simulink model "untitled_restored_from_autosave"  (R2020a)
settings: Solver=VariableStepAuto  StartTime=0.0  StopTime=0.0  RelTol=1e-3
(part 2 of 2)

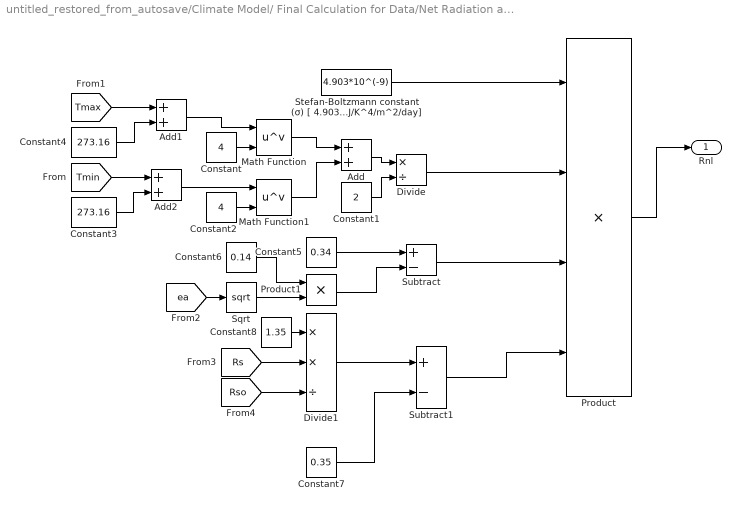
== system untitled_restored_from_autosave/Climate Model/ Final Calculation for Data/Net Radiation at the Crop Surface (Rn) [MJ//m^2//day]/Net Longwave Radiation (Rnl) [MJ//m^2//day] ==
  Add : Sum
  Add1 : Sum
  Add2 : Sum
  Constant : Constant  Value=4
  Constant1 : Constant  Value=2
  Constant2 : Constant  Value=4
  Constant3 : Constant  Value=273.16
  Constant4 : Constant  Value=273.16
  Constant5 : Constant  Value=0.34
  Constant6 : Constant  Value=0.14
  Constant7 : Constant  Value=0.35
  Constant8 : Constant  Value=1.35
  Divide : Product  Inputs=*/
  Divide1 : Product  Inputs=**/
  Math Function : Math  Operator=pow  SaturateOnIntegerOverflow=on
  Math Function1 : Math  Operator=pow  SaturateOnIntegerOverflow=on
  Product : Product  Inputs=4
  Product1 : Product
  Sqrt : Sqrt  SaturateOnIntegerOverflow=on
  Stefan-Boltzmann constant (σ) [ 4.903 10^-9 MJ/K^4/m^2/day] : Constant  Value=4.903*10^(-9)
  Subtract : Sum  Inputs=+-
  Subtract1 : Sum  Inputs=+-
  Rnl : Outport
  wires:
  Product/1 -> Rnl/1
  Stefan-Boltzmann constant (σ) [ 4.903 10^-9 MJ/K^4/m^2/day]/1 -> Product/1
  Constant/1 -> Math Function/2
  Math Function/1 -> Add/1
  Add/1 -> Divide/1
  Divide/1 -> Product/2
  Constant1/1 -> Divide/2
  Math Function1/1 -> Add/2
  Constant2/1 -> Math Function1/2
  Add1/1 -> Math Function/1
  Add2/1 -> Math Function1/1
  Constant3/1 -> Add2/2
  Constant4/1 -> Add1/2
  [Tmin] -> Add2/1
  [Tmax] -> Add1/1
  Subtract/1 -> Product/3
  Constant5/1 -> Subtract/1
  Product1/1 -> Subtract/2
  Constant6/1 -> Product1/1
  Sqrt/1 -> Product1/2
  [ea] -> Sqrt/1
  Subtract1/1 -> Product/4
  Divide1/1 -> Subtract1/1
  Constant7/1 -> Subtract1/2
  Constant8/1 -> Divide1/1
  [Rso] -> Divide1/3
  [Rs] -> Divide1/2

== system untitled_restored_from_autosave/Climate Model/ Final Calculation for Data/Net Radiation at the Crop Surface (Rn) [MJ//m^2//day]/Net Solar//Shortwave Radiation (Rns) [MJ//m^2//day] ==
  Albedo or canopy reflection coefficient for the reference crop (G) : Subsystem
  Constant : Constant
  Product : Product
  Subtract : Sum  Inputs=+-
  Out1 : Outport
  wires:
  Product/1 -> Out1/1
  Constant/1 -> Subtract/1
  Albedo or canopy reflection coefficient for the reference crop (G)/1(Out1) -> Subtract/2
  Subtract/1 -> Product/1
  [Rs] -> Product/2

== system untitled_restored_from_autosave/Climate Model/ Final Calculation for Data/Net Radiation at the Crop Surface (Rn) [MJ//m^2//day]/Solar Radiation (Rs) [MJ//m^2//day] ==
  Actual Duration of Sunlight (n) [hour] : Constant  Value=12
  Angstrom Formula if AI_Rs not avaliable : Subsystem
  Constant : Constant  Value=Ac_Rs
  Constant1 : Constant  Value=5
  Hargreaves Formula if AI_Rs and hour of daylight is not available : Subsystem  mask{kRs=0.16}
      mask prompts: kRs "Adjustment Coefficient"
      mask DialogControl Control2 Prompt: The square root of the temperature difference is closely related to the existing daily solar radiation in a given location. The adjustment coefficient kRs is empirical and differs for 'interior' or 'coastal' regions:
      mask DialogControl Control3 Prompt: · for 'interior' locations, where land mass dominates and air masses are not strongly influenced by a large water body, kRs @ 0.16;
      mask DialogControl Control4 Prompt: · for 'coastal' locations, situated on or adjacent to the coast of a large land mass and where air masses are influenced by a nearby water body, kRs @ 0.19.
  Index Vector : MultiPortSwitch
  Rs : Outport
  wires:
  Constant/1 -> Index Vector/1
  Constant1/1 -> Index Vector/2
  Angstrom Formula if AI_Rs not avaliable/1(Out1) -> Index Vector/3
  Index Vector/1 -> Rs/1
  Hargreaves Formula if AI_Rs and hour of daylight is not available/1(Rs) -> Index Vector/4
  Actual Duration of Sunlight (n) [hour]/1 -> Angstrom Formula if AI_Rs not avaliable/1(In1)

== system untitled_restored_from_autosave/Climate Model/ Final Calculation for Data/Wind Speed/Wind Speed measured at 2m height (u2) [m//s] ==
  uz : Inport
  z : Inport  Port=2
  Constant : Constant  Value=4.87
  Constant1 : Constant  Value=67.8
  Constant2 : Constant  Value=5.42
  Divide : Product  Inputs=**/
  Math Function : Math  Operator=log  SaturateOnIntegerOverflow=on
  Product : Product
  Subtract : Sum  Inputs=+-
  u2 : Outport
  wires:
  uz/1 -> Divide/1
  Constant/1 -> Divide/2
  Math Function/1 -> Divide/3
  z/1 -> Product/2
  Constant1/1 -> Product/1
  Product/1 -> Subtract/1
  Subtract/1 -> Math Function/1
  Constant2/1 -> Subtract/2
  Divide/1 -> u2/1

== system untitled_restored_from_autosave/Estimated Soil Heat Capacity (UC Davis)/Bulk Density (Saxton and Rawls Function) [g//cm^3)/Normal Density (g//cm^3)/Saturated Moisture θS ==
  Constant : Constant  Value=0.097
  Constant1 : Constant  Value=0.043
  Product : Product
  Subtract : Sum  Inputs=++-+
  θ(S-33) : Subsystem
  Out1 : Outport
  wires:
  Subtract/1 -> Out1/1
  [qFC] -> Subtract/1
  Product/1 -> Subtract/3
  Constant/1 -> Product/1
  [PSand] -> Product/2
  Constant1/1 -> Subtract/4
  θ(S-33)/1(Out1) -> Subtract/2

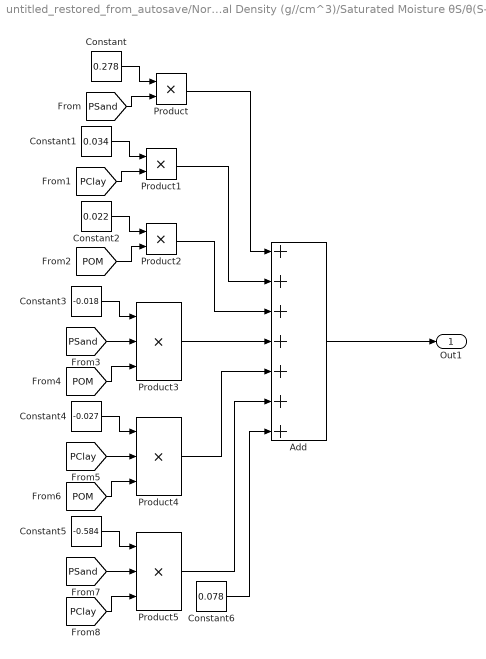
== system untitled_restored_from_autosave/Normal Density (g//cm^3)/Saturated Moisture θS/θ(S-33)/θ(S-33)t ==
  Add : Sum  Inputs=+++++++
  Constant : Constant  Value=0.278
  Constant1 : Constant  Value=0.034
  Constant2 : Constant  Value=0.022
  Constant3 : Constant  Value=-0.018
  Constant4 : Constant  Value=-0.027
  Constant5 : Constant  Value=-0.584
  Constant6 : Constant  Value=0.078
  Product : Product
  Product1 : Product
  Product2 : Product
  Product3 : Product  Inputs=3
  Product4 : Product  Inputs=3
  Product5 : Product  Inputs=3
  Out1 : Outport
  wires:
  Add/1 -> Out1/1
  Constant2/1 -> Product2/1
  [POM] -> Product2/2
  Product1/1 -> Add/2
  Product2/1 -> Add/3
  [PClay] -> Product4/2
  Constant3/1 -> Product3/1
  [POM] -> Product3/3
  [PClay] -> Product1/2
  Constant6/1 -> Add/7
  Product5/1 -> Add/6
  [PClay] -> Product5/3
  Product/1 -> Add/1
  Constant5/1 -> Product5/1
  Constant1/1 -> Product1/1
  Constant/1 -> Product/1
  [POM] -> Product4/3
  Product3/1 -> Add/4
  [PSand] -> Product5/2
  [PSand] -> Product3/2
  Constant4/1 -> Product4/1
  [PSand] -> Product/2
  Product4/1 -> Add/5

== system untitled_restored_from_autosave/Reference Evapotraspiration (ET0) [mm//day]/Actual Vapor Pressure (ea) [kPa]/Derived from Dewpoint Temperature/Saturation Vapor Pressure (eo) ==
  In1 : Inport
  Add : Sum
  Constant : Constant  Value=0.6108
  Constant1 : Constant  Value=17.27
  Constant2 : Constant  Value=237.3
  Divide : Product  Inputs=**/
  Math Function : Math  SaturateOnIntegerOverflow=on
  Product : Product
  Out1 : Outport
  wires:
  Product/1 -> Out1/1
  Constant1/1 -> Divide/1
  In1/1 -> Add/1, Divide/2
  Add/1 -> Divide/3
  Divide/1 -> Math Function/1
  Constant/1 -> Product/1
  Constant2/1 -> Add/2
  Math Function/1 -> Product/2

== system untitled_restored_from_autosave/Reference Evapotraspiration (ET0) [mm//day]/Actual Vapor Pressure (ea) [kPa]/Derived from Psychrometric Data/Saturation Vapor Pressure (eo) ==
  In1 : Inport
  Add : Sum
  Constant : Constant  Value=0.6108
  Constant1 : Constant  Value=17.27
  Constant2 : Constant  Value=237.3
  Divide : Product  Inputs=**/
  Math Function : Math  SaturateOnIntegerOverflow=on
  Product : Product
  Out1 : Outport
  wires:
  Product/1 -> Out1/1
  Constant1/1 -> Divide/1
  In1/1 -> Add/1, Divide/2
  Add/1 -> Divide/3
  Divide/1 -> Math Function/1
  Constant/1 -> Product/1
  Constant2/1 -> Add/2
  Math Function/1 -> Product/2

== system untitled_restored_from_autosave/Reference Evapotraspiration (ET0) [mm//day]/Actual Vapor Pressure (ea) [kPa]/Derived from RHmax & RHmin/Saturation Vapor Pressure (eo) ==
  In1 : Inport
  Add : Sum
  Constant : Constant  Value=0.6108
  Constant1 : Constant  Value=17.27
  Constant2 : Constant  Value=237.3
  Divide : Product  Inputs=**/
  Math Function : Math  SaturateOnIntegerOverflow=on
  Product : Product
  Out1 : Outport
  wires:
  Product/1 -> Out1/1
  Constant1/1 -> Divide/1
  In1/1 -> Add/1, Divide/2
  Add/1 -> Divide/3
  Divide/1 -> Math Function/1
  Constant/1 -> Product/1
  Constant2/1 -> Add/2
  Math Function/1 -> Product/2

== system untitled_restored_from_autosave/Reference Evapotraspiration (ET0) [mm//day]/Actual Vapor Pressure (ea) [kPa]/Derived from RHmax & RHmin/Saturation Vapor Pressure (eo)1 ==
  In1 : Inport
  Add : Sum
  Constant : Constant  Value=0.6108
  Constant1 : Constant  Value=17.27
  Constant2 : Constant  Value=237.3
  Divide : Product  Inputs=**/
  Math Function : Math  SaturateOnIntegerOverflow=on
  Product : Product
  Out1 : Outport
  wires:
  Math Function/1 -> Product/2
  Constant2/1 -> Add/2
  Constant/1 -> Product/1
  Divide/1 -> Math Function/1
  Add/1 -> Divide/3
  In1/1 -> Divide/2, Add/1
  Constant1/1 -> Divide/1
  Product/1 -> Out1/1

== system untitled_restored_from_autosave/Reference Evapotraspiration (ET0) [mm//day]/Actual Vapor Pressure (ea) [kPa]/Derived from RHmax only/Saturation Vapor Pressure (eo) ==
  In1 : Inport
  Add : Sum
  Constant : Constant  Value=0.6108
  Constant1 : Constant  Value=17.27
  Constant2 : Constant  Value=237.3
  Divide : Product  Inputs=**/
  Math Function : Math  SaturateOnIntegerOverflow=on
  Product : Product
  Out1 : Outport
  wires:
  Product/1 -> Out1/1
  Constant1/1 -> Divide/1
  In1/1 -> Add/1, Divide/2
  Add/1 -> Divide/3
  Divide/1 -> Math Function/1
  Constant/1 -> Product/1
  Constant2/1 -> Add/2
  Math Function/1 -> Product/2

== system untitled_restored_from_autosave/Reference Evapotraspiration (ET0) [mm//day]/Actual Vapor Pressure (ea) [kPa]/Derived from RHmean only/Saturation Vapor Pressure (eo) ==
  In1 : Inport
  Add : Sum
  Constant : Constant  Value=0.6108
  Constant1 : Constant  Value=17.27
  Constant2 : Constant  Value=237.3
  Divide : Product  Inputs=**/
  Math Function : Math  SaturateOnIntegerOverflow=on
  Product : Product
  Out1 : Outport
  wires:
  Product/1 -> Out1/1
  Constant1/1 -> Divide/1
  In1/1 -> Add/1, Divide/2
  Add/1 -> Divide/3
  Divide/1 -> Math Function/1
  Constant/1 -> Product/1
  Constant2/1 -> Add/2
  Math Function/1 -> Product/2

== system untitled_restored_from_autosave/Reference Evapotraspiration (ET0) [mm//day]/Actual Vapor Pressure (ea) [kPa]/Derived from RHmean only/Saturation Vapor Pressure (eo)1 ==
  In1 : Inport
  Add : Sum
  Constant : Constant  Value=0.6108
  Constant1 : Constant  Value=17.27
  Constant2 : Constant  Value=237.3
  Divide : Product  Inputs=**/
  Math Function : Math  SaturateOnIntegerOverflow=on
  Product : Product
  Out1 : Outport
  wires:
  Math Function/1 -> Product/2
  Constant2/1 -> Add/2
  Constant/1 -> Product/1
  Divide/1 -> Math Function/1
  Add/1 -> Divide/3
  In1/1 -> Divide/2, Add/1
  Constant1/1 -> Divide/1
  Product/1 -> Out1/1

== system untitled_restored_from_autosave/Soil Data Calculation/Estimated Soil Heat Capacity (UC Davis)/Bulk Density (Saxton and Rawls Function) [g//cm^3)/Normal Density (g//cm^3) ==
  Constant : Constant  Value=2.65
  Constant1 : Constant
  Product : Product
  Saturated Moisture θS : Subsystem
  Subtract : Sum  Inputs=+-
  Out1 : Outport
  wires:
  Product/1 -> Out1/1
  Constant/1 -> Product/2
  Subtract/1 -> Product/1
  Constant1/1 -> Subtract/1
  Saturated Moisture θS/1(Out1) -> Subtract/2

== system untitled_restored_from_autosave/Soil Data Calculation/Estimated Soil Heat Capacity (UC Davis)/Bulk Density (Saxton and Rawls Function) [g//cm^3)/Volum Fraction of Gravel (g//cm^3) ==
  In1 : Inport
  Constant : Constant  Value=2.65
  Constant1 : Constant
  Constant2 : Constant
  Divide : Product  Inputs=*/
  Divide1 : Product  Inputs=*/
  Product : Product
  Product1 : Product
  Subtract : Sum  Inputs=+-
  Subtract1 : Sum  Inputs=+-
  Out1 : Outport
  wires:
  In1/1 -> Divide/1
  [PGravel] -> Product1/1, Product/2
  Constant/1 -> Divide/2
  Divide/1 -> Subtract1/2, Product/1
  Product/1 -> Divide1/1
  Subtract/1 -> Divide1/2
  Constant1/1 -> Subtract/1
  Product1/1 -> Subtract/2
  Subtract1/1 -> Product1/2
  Constant2/1 -> Subtract1/1
  Divide1/1 -> Out1/1

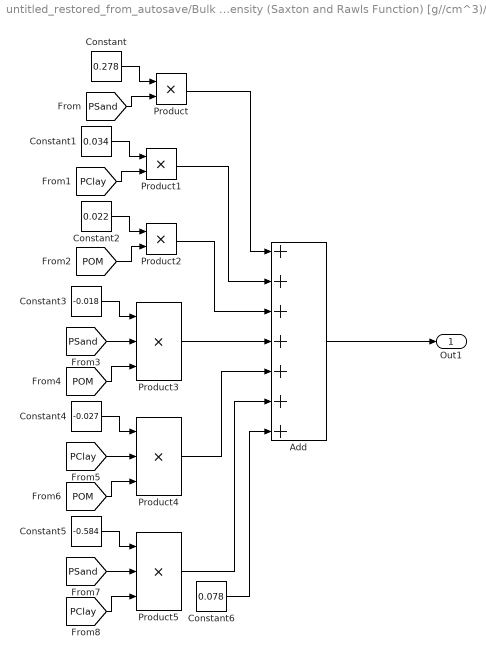
== system untitled_restored_from_autosave/Bulk Density (Saxton and Rawls Function) [g//cm^3)/Normal Density (g//cm^3)/Saturated Moisture θS/θ(S-33)/θ(S-33)t ==
  Add : Sum  Inputs=+++++++
  Constant : Constant  Value=0.278
  Constant1 : Constant  Value=0.034
  Constant2 : Constant  Value=0.022
  Constant3 : Constant  Value=-0.018
  Constant4 : Constant  Value=-0.027
  Constant5 : Constant  Value=-0.584
  Constant6 : Constant  Value=0.078
  Product : Product
  Product1 : Product
  Product2 : Product
  Product3 : Product  Inputs=3
  Product4 : Product  Inputs=3
  Product5 : Product  Inputs=3
  Out1 : Outport
  wires:
  Add/1 -> Out1/1
  Constant2/1 -> Product2/1
  [POM] -> Product2/2
  Product1/1 -> Add/2
  Product2/1 -> Add/3
  [PClay] -> Product4/2
  Constant3/1 -> Product3/1
  [POM] -> Product3/3
  [PClay] -> Product1/2
  Constant6/1 -> Add/7
  Product5/1 -> Add/6
  [PClay] -> Product5/3
  Product/1 -> Add/1
  Constant5/1 -> Product5/1
  Constant1/1 -> Product1/1
  Constant/1 -> Product/1
  [POM] -> Product4/3
  Product3/1 -> Add/4
  [PSand] -> Product5/2
  [PSand] -> Product3/2
  Constant4/1 -> Product4/1
  [PSand] -> Product/2
  Product4/1 -> Add/5

== system untitled_restored_from_autosave/Climate Model/ Final Calculation for Data/Net Radiation at the Crop Surface (Rn) [MJ//m^2//day]/Extraterrestrial Radiation (Ra) [MJ//m^2//day]/Inverse Relative Distance Earth-Sun (dr) ==
  J : Inport
  Add : Sum
  Constant : Constant
  Constant1 : Constant  Value=0.033
  Constant2 : Constant  Value=2*pi
  Divide : Product  Inputs=**/
  Product : Product
  Trigonometric Function : Trigonometry  Operator=cos
  dr : Outport
  wires:
  Add/1 -> dr/1
  Constant/1 -> Add/1
  Product/1 -> Add/2
  Constant1/1 -> Product/1
  Trigonometric Function/1 -> Product/2
  Divide/1 -> Trigonometric Function/1
  Constant2/1 -> Divide/1
  [DinYear] -> Divide/3
  J/1 -> Divide/2

== system untitled_restored_from_autosave/Climate Model/ Final Calculation for Data/Net Radiation at the Crop Surface (Rn) [MJ//m^2//day]/Extraterrestrial Radiation (Ra) [MJ//m^2//day]/Latitude in Radian (φ) [rad] ==
  Add : Sum
  Constant : Constant  Value=pi/180
  Constant1 : Constant  Value=60
  Divide : Product  Inputs=*/
  Product : Product
  φ : Outport
  wires:
  Constant/1 -> Product/1
  Add/1 -> Product/2
  [LatDeg] -> Add/1
  [LatMin] -> Divide/1
  Constant1/1 -> Divide/2
  Divide/1 -> Add/2
  Product/1 -> φ/1

== system untitled_restored_from_autosave/Climate Model/ Final Calculation for Data/Net Radiation at the Crop Surface (Rn) [MJ//m^2//day]/Extraterrestrial Radiation (Ra) [MJ//m^2//day]/Solar Declination in Radian (δ) [rad] ==
  J : Inport
  Constant1 : Constant  Value=0.409
  Constant2 : Constant  Value=2*pi
  Constant4 : Constant  Value=1.39
  Divide : Product  Inputs=**/
  Product : Product
  Subtract : Sum  Inputs=+-
  Trigonometric Function : Trigonometry
  δ : Outport
  wires:
  [DinYear] -> Divide/3
  Product/1 -> δ/1
  Trigonometric Function/1 -> Product/2
  J/1 -> Divide/2
  Constant2/1 -> Divide/1
  Constant1/1 -> Product/1
  Divide/1 -> Subtract/1
  Subtract/1 -> Trigonometric Function/1
  Constant4/1 -> Subtract/2

== system untitled_restored_from_autosave/Climate Model/ Final Calculation for Data/Net Radiation at the Crop Surface (Rn) [MJ//m^2//day]/Extraterrestrial Radiation (Ra) [MJ//m^2//day]/Sunset Hour Angle (Ws) [rad] ==
  Constant : Constant  Value=-1
  Product : Product  Inputs=3
  Trigonometric Function : Trigonometry  Operator=acos
  Trigonometric Function1 : Trigonometry  Operator=tan
  Trigonometric Function2 : Trigonometry  Operator=tan
  Ws : Outport
  wires:
  Trigonometric Function/1 -> Ws/1
  Product/1 -> Trigonometric Function/1
  Constant/1 -> Product/1
  Trigonometric Function1/1 -> Product/2
  Trigonometric Function2/1 -> Product/3
  [LatRad] -> Trigonometric Function1/1
  [SolDec] -> Trigonometric Function2/1

== system untitled_restored_from_autosave/Climate Model/ Final Calculation for Data/Net Radiation at the Crop Surface (Rn) [MJ//m^2//day]/Net Solar//Shortwave Radiation (Rns) [MJ//m^2//day]/Albedo or canopy reflection coefficient for the reference crop (G) ==
  Constant : Constant  Value=0.23
  Out1 : Outport
  wires:
  Constant/1 -> Out1/1

== system untitled_restored_from_autosave/Climate Model/ Final Calculation for Data/Net Radiation at the Crop Surface (Rn) [MJ//m^2//day]/Solar Radiation (Rs) [MJ//m^2//day]/Angstrom Formula if AI_Rs not avaliable ==
  In1 : Inport
  Add : Sum
  Default as : Constant  Value=0.25
  Default bs : Constant  Value=0.50
  Divide : Product  Inputs=**/
  Maximum Daylight Hour (N) [hour] : Subsystem
  Product : Product
  Out1 : Outport
  wires:
  Default as/1 -> Add/1
  Default bs/1 -> Divide/1
  Divide/1 -> Add/2
  In1/1 -> Divide/2
  Add/1 -> Product/1
  Product/1 -> Out1/1
  [Ra] -> Product/2
  Maximum Daylight Hour (N) [hour]/1(N) -> Divide/3

== system untitled_restored_from_autosave/Climate Model/ Final Calculation for Data/Net Radiation at the Crop Surface (Rn) [MJ//m^2//day]/Solar Radiation (Rs) [MJ//m^2//day]/Hargreaves Formula if AI_Rs and hour of daylight is not available ==
  Constant : Constant  Value=kRs
  Product : Product  Inputs=3
  Sqrt : Sqrt  SaturateOnIntegerOverflow=on
  Subtract : Sum  Inputs=+-
  Rs : Outport
  wires:
  Product/1 -> Rs/1
  Constant/1 -> Product/1
  [Ra] -> Product/3
  Sqrt/1 -> Product/2
  Subtract/1 -> Sqrt/1
  [Tmin] -> Subtract/2
  [Tmax] -> Subtract/1

== system untitled_restored_from_autosave/Estimated Soil Heat Capacity (UC Davis)/Bulk Density (Saxton and Rawls Function) [g//cm^3)/Normal Density (g//cm^3)/Saturated Moisture θS/θ(S-33) ==
  Constant : Constant  Value=0.636
  Constant1 : Constant  Value=0.107
  Product : Product
  Subtract : Sum  Inputs=++-
  θ(S-33)t : Subsystem
  Out1 : Outport
  wires:
  θ(S-33)t/1(Out1) -> Product/1, Subtract/1
  Product/1 -> Subtract/2
  Constant/1 -> Product/2
  Constant1/1 -> Subtract/3
  Subtract/1 -> Out1/1

== system untitled_restored_from_autosave/Soil Data Calculation/Estimated Soil Heat Capacity (UC Davis)/Bulk Density (Saxton and Rawls Function) [g//cm^3)/Normal Density (g//cm^3)/Saturated Moisture θS ==
  Constant : Constant  Value=0.097
  Constant1 : Constant  Value=0.043
  Product : Product
  Subtract : Sum  Inputs=++-+
  θ(S-33) : Subsystem
  Out1 : Outport
  wires:
  Subtract/1 -> Out1/1
  [qFC] -> Subtract/1
  Product/1 -> Subtract/3
  Constant/1 -> Product/1
  [PSand] -> Product/2
  Constant1/1 -> Subtract/4
  θ(S-33)/1(Out1) -> Subtract/2

== system untitled_restored_from_autosave/Climate Model/ Final Calculation for Data/Net Radiation at the Crop Surface (Rn) [MJ//m^2//day]/Solar Radiation (Rs) [MJ//m^2//day]/Angstrom Formula if AI_Rs not avaliable/Maximum Daylight Hour (N) [hour] ==
  Constant : Constant  Value=24
  Constant1 : Constant  Value=pi
  Divide : Product  Inputs=**/
  N : Outport
  wires:
  Divide/1 -> N/1
  [Ws] -> Divide/2
  Constant/1 -> Divide/1
  Constant1/1 -> Divide/3

== system untitled_restored_from_autosave/Estimated Soil Heat Capacity (UC Davis)/Bulk Density (Saxton and Rawls Function) [g//cm^3)/Normal Density (g//cm^3)/Saturated Moisture θS/θ(S-33)/θ(S-33)t ==
  Add : Sum  Inputs=+++++++
  Constant : Constant  Value=0.278
  Constant1 : Constant  Value=0.034
  Constant2 : Constant  Value=0.022
  Constant3 : Constant  Value=-0.018
  Constant4 : Constant  Value=-0.027
  Constant5 : Constant  Value=-0.584
  Constant6 : Constant  Value=0.078
  Product : Product
  Product1 : Product
  Product2 : Product
  Product3 : Product  Inputs=3
  Product4 : Product  Inputs=3
  Product5 : Product  Inputs=3
  Out1 : Outport
  wires:
  Add/1 -> Out1/1
  Constant2/1 -> Product2/1
  [POM] -> Product2/2
  Product1/1 -> Add/2
  Product2/1 -> Add/3
  [PClay] -> Product4/2
  Constant3/1 -> Product3/1
  [POM] -> Product3/3
  [PClay] -> Product1/2
  Constant6/1 -> Add/7
  Product5/1 -> Add/6
  [PClay] -> Product5/3
  Product/1 -> Add/1
  Constant5/1 -> Product5/1
  Constant1/1 -> Product1/1
  Constant/1 -> Product/1
  [POM] -> Product4/3
  Product3/1 -> Add/4
  [PSand] -> Product5/2
  [PSand] -> Product3/2
  Constant4/1 -> Product4/1
  [PSand] -> Product/2
  Product4/1 -> Add/5

== system untitled_restored_from_autosave/Soil Data Calculation/Estimated Soil Heat Capacity (UC Davis)/Bulk Density (Saxton and Rawls Function) [g//cm^3)/Normal Density (g//cm^3)/Saturated Moisture θS/θ(S-33) ==
  Constant : Constant  Value=0.636
  Constant1 : Constant  Value=0.107
  Product : Product
  Subtract : Sum  Inputs=++-
  θ(S-33)t : Subsystem
  Out1 : Outport
  wires:
  θ(S-33)t/1(Out1) -> Product/1, Subtract/1
  Product/1 -> Subtract/2
  Constant/1 -> Product/2
  Constant1/1 -> Subtract/3
  Subtract/1 -> Out1/1

== system untitled_restored_from_autosave/Soil Data Calculation/Estimated Soil Heat Capacity (UC Davis)/Bulk Density (Saxton and Rawls Function) [g//cm^3)/Normal Density (g//cm^3)/Saturated Moisture θS/θ(S-33)/θ(S-33)t ==
  Add : Sum  Inputs=+++++++
  Constant : Constant  Value=0.278
  Constant1 : Constant  Value=0.034
  Constant2 : Constant  Value=0.022
  Constant3 : Constant  Value=-0.018
  Constant4 : Constant  Value=-0.027
  Constant5 : Constant  Value=-0.584
  Constant6 : Constant  Value=0.078
  Product : Product
  Product1 : Product
  Product2 : Product
  Product3 : Product  Inputs=3
  Product4 : Product  Inputs=3
  Product5 : Product  Inputs=3
  Out1 : Outport
  wires:
  Add/1 -> Out1/1
  Constant2/1 -> Product2/1
  [POM] -> Product2/2
  Product1/1 -> Add/2
  Product2/1 -> Add/3
  [PClay] -> Product4/2
  Constant3/1 -> Product3/1
  [POM] -> Product3/3
  [PClay] -> Product1/2
  Constant6/1 -> Add/7
  Product5/1 -> Add/6
  [PClay] -> Product5/3
  Product/1 -> Add/1
  Constant5/1 -> Product5/1
  Constant1/1 -> Product1/1
  Constant/1 -> Product/1
  [POM] -> Product4/3
  Product3/1 -> Add/4
  [PSand] -> Product5/2
  [PSand] -> Product3/2
  Constant4/1 -> Product4/1
  [PSand] -> Product/2
  Product4/1 -> Add/5

== matlab function untitled_restored_from_autosave/Plant Model/General Plant Database/MATLAB Function1 ==
  data: PDd input; cd output; PDm input; PDy input; DafterPD input; d output; m output; y output
function [cd,d,m,y] = curDate(PDd,PDm,PDy,DafterPD)
    x = datetime(PDy,PDm,PDd);
    x = x + floor(DafterPD);
    xv = datevec(x);
    y = xv(1);
    m = xv(2);
    d = xv(3);
    xm = datetime(y,1,1);
    a = minus(x,xm);
    cd = days(a);
end

== matlab function untitled_restored_from_autosave/Plant Model/General Plant Database/MATLAB Function ==
  data: year input; D output
function D = DinYear(year)
    if mod(year, 4) == 0
        D = 366;
        if mod(year, 100) == 0
            D = 365;
            if mod(year,400)==0
                D = 366;
            end
        end
    else
        D = 365;
    end
end

== matlab function untitled_restored_from_autosave/Plant Model/Plant Data Calculation/MATLAB Function ==
  data: d input; stage output; Lini input; Ldev input; Lmid input; Llate input
function stage = curPS(d,Lini,Ldev,Lmid,Llate)
    stage = 0;
    d = d - Lini;
    if d <= 0
        return
    end
    stage = 1;
    d = d - Ldev;
    if d <= 0
        return
    end
    stage = 2;
    d = d - Lmid;
    if d <= 0
        return
    end
    stage = 3;
    d = d - Lmid;
    if d <= 0 
        return
    end
    stage = 4;
end

== matlab function untitled_restored_from_autosave/General Soil Database/MATLAB Function3 ==
  data: sand input; clay input; orgmat input; SC output; sand output; silt output; clay output; orgmat output; CMF output
function [SC,sand, silt, clay, orgmat, CMF] = soil_classification(sand, clay, orgmat)

 if sand>1
     sand=sand/100;
 end
 if orgmat>1
     orgmat=orgmat/100;
 end
 if clay>1
     clay=clay/100;
 end
 if (sand + orgmat + clay > 1) || sand<0 || clay<0 || orgmat<0
    error('data inconsisent: soil compositions need to sum to 1')
 end
%--------------------------------------------------------------------------
%--------------------------------------------------------------------------
%--------------------------------------------------------------------------
silt = 1 - sand - clay - orgmat;
if (silt+1.5*clay)<.15
     SC ="SAND";
     CMF = 1;
 elseif ((silt+1.5*clay)>=.15)&&((silt+2*clay)<.3)
     SC ="LOAMY SAND";
     CMF = 1;
 elseif (clay>=0.07) && (clay<=0.2) && (sand>0.52) && ((silt+2*clay)>=0.3) 
     SC ="SANDY LOAM";
     CMF = 1;
 elseif (clay<0.07) && (silt < 0.5) && ((silt+2*clay)>=0.3)
     SC ="SANDY LOAM";
     CMF = 1;
 elseif (clay>=0.07) && (clay<=0.27) && (silt>=0.28) && (silt<0.5) && (sand<=0.52)
     SC ="LOAM";
     CMF = 2;
 elseif ((silt>=0.5) && clay>=0.12 && clay<0.27) || (silt>=0.5 && silt<0.8 && clay<0.12)
     SC ="SILT LOAM";
     CMF = 2;
 elseif silt>=0.8 && clay<0.12
     SC ="SILT";
     CMF = 2;
 elseif clay>=0.2 && clay<0.35 && silt<0.28 && sand>0.45
     SC ="SANDY CLAY LOAM";
     CMF = 2;
 elseif clay>=0.27 && clay <0.4 && sand>0.2 && sand<=0.45
     SC ="CLAY LOAM";
     CMF = 3;
 elseif clay>=0.27 && clay<0.4 && sand<=0.2
     SC ="SILTY CLAY LOAM";
     CMF = 3;
 elseif clay>=0.35 && sand>=0.45
     SC ="SANDY CLAY";
     CMF = 3;
 elseif clay>=0.4 && silt>=0.4
     SC ="SILTY CLAY";
     CMF = 3;
 elseif clay>= 0.4 && sand<=0.45 && silt<0.4
     SC ="CLAY";
     CMF = 3;
 else
     error('no soil class found')
end
end %of function
